simulink model "Motor"  (R2016b)
settings: Solver=FixedStepAuto  StartTime=0.0  StopTime=10.0  RelTol=1e-3
settings Model: Creator=NEATdemo  LastModifiedBy=NEATdemo

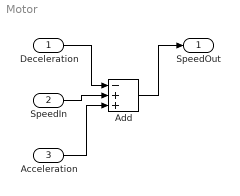
== system Motor ==
  Deceleration : Inport
      settings: AttributesFormatString=speed
  SpeedIn : Inport  Port=2
      settings: AttributesFormatString=speed
  Acceleration : Inport  Port=3
      settings: AttributesFormatString=speed
  Add : Sum  Inputs=-++
  SpeedOut : Outport
      settings: AttributesFormatString=speed
  wires:
  Deceleration/1 -> Add/1
  SpeedIn/1 -> Add/2
  Acceleration/1 -> Add/3
  Add/1 -> SpeedOut/1
